simulink model "Clutch"  (R2020a)
settings: Solver=VariableStepAuto  StartTime=0.0  StopTime=10.0  RelTol=1e-3
undefined symbols (not defined in the file or in its folder): be, bv, Ie, Iv, R, uk, us
settings Model: DataDictionary=Clutch_lockup.sldd  Creator=USER  LastModifiedBy=USER

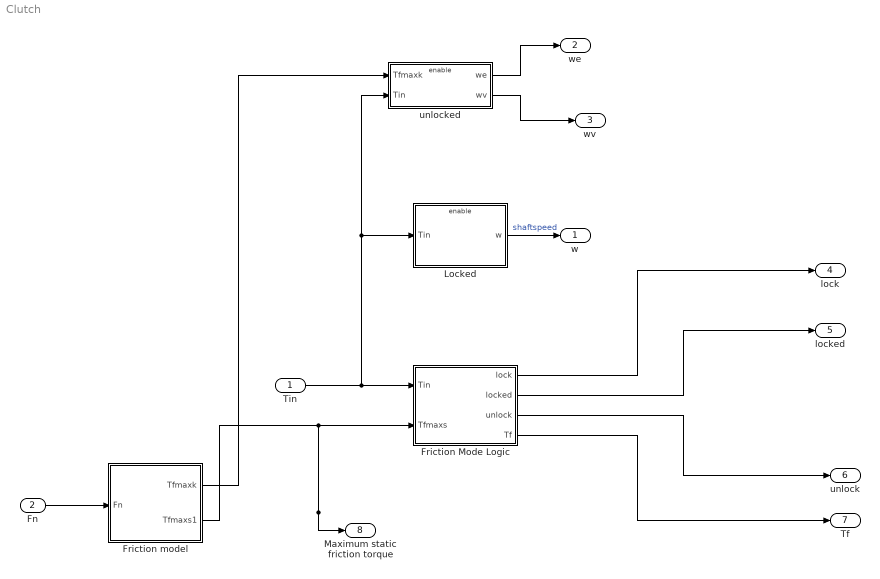
== system Clutch ==
  Tin : Inport
  Fn : Inport  Port=2
  Friction Mode Logic : Subsystem
  Friction model : Subsystem
  Locked : Subsystem
  unlocked : Subsystem
  w : Outport
  we : Outport  Port=2
  wv : Outport  Port=3
  lock : Outport  Port=4
  locked : Outport  Port=5
  unlock : Outport  Port=6
  Tf : Outport  Port=7
  Maximum static friction torque : Outport  Port=8
  wires:
  Locked/1(w) -> w/1  "shaftspeed"
  unlocked/1(we) -> we/1
  unlocked/2(wv) -> wv/1
  Friction model/2(Tfmaxs1) -> Maximum static friction torque/1, Friction Mode Logic/2(Tfmaxs)
  Tin/1 -> unlocked/2(Tin), Locked/1(Tin), Friction Mode Logic/1(Tin)
  Friction Mode Logic/1(lock) -> lock/1
  Friction Mode Logic/2(locked) -> locked/1
  Friction Mode Logic/3(unlock) -> unlock/1
  Friction Mode Logic/4(Tf) -> Tf/1
  Fn/1 -> Friction model/1(Fn)
  Friction model/1(Tfmaxk) -> unlocked/1(Tfmaxk)

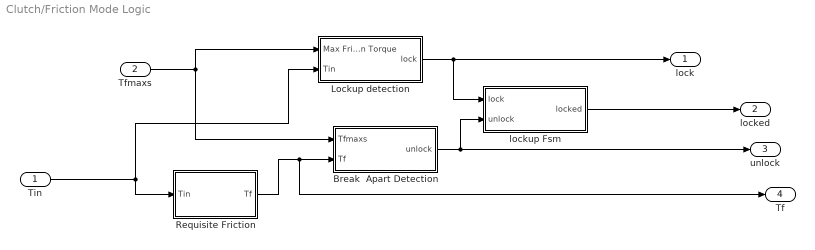
== system Clutch/Friction Mode Logic ==
  Tin : Inport
  Tfmaxs : Inport  Port=2
  Break  Apart Detection : Subsystem
  Lockup detection : Subsystem
  Requisite Friction : Subsystem
  lockup Fsm : Subsystem
  lock : Outport
  locked : Outport  Port=2
  unlock : Outport  Port=3
  Tf : Outport  Port=4
  wires:
  Lockup detection/1(lock) -> lock/1, lockup Fsm/1(lock)
  Requisite Friction/1(Tf) -> Tf/1, Break  Apart Detection/2(Tf)
  Tin/1 -> Lockup detection/2(Tin), Requisite Friction/1(Tin)
  Break  Apart Detection/1(unlock) -> unlock/1, lockup Fsm/2(unlock)
  Tfmaxs/1 -> Break  Apart Detection/1(Tfmaxs), Lockup detection/1(Max Friction Torque)
  lockup Fsm/1(locked) -> locked/1

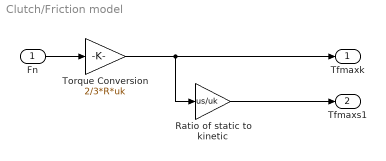
== system Clutch/Friction model ==
  Fn : Inport
  Ratio of static to kinetic : Gain  Gain=us/uk  SaturateOnIntegerOverflow=on  OutDataTypeStr=Inherit: Same as input  ParamDataTypeStr=Inherit: Same as input
  Torque Conversion : Gain  Gain=2/3*R*uk  SaturateOnIntegerOverflow=on  OutDataTypeStr=Inherit: Same as input  ParamDataTypeStr=Inherit: Same as input
  Tfmaxk : Outport  InitialOutput=0  VectorParamsAs1DForOutWhenUnconnected=off
  Tfmaxs1 : Outport  Port=2  InitialOutput=0  VectorParamsAs1DForOutWhenUnconnected=off
  wires:
  Torque Conversion/1 -> Tfmaxk/1, Ratio of static to kinetic/1
  Ratio of static to kinetic/1 -> Tfmaxs1/1
  Fn/1 -> Torque Conversion/1

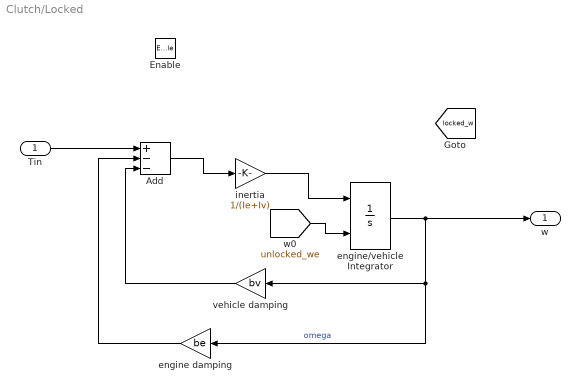
== system Clutch/Locked ==
  Tin : Inport
  Enable : EnablePort  StatesWhenEnabling=reset
  Add : Sum  Inputs=+--
  engine damping : Gain  Gain=be
  engine/vehicle Integrator : Integrator  InitialConditionSource=external
  inertia : Gain  Gain=1/(Ie+Iv)
  vehicle damping : Gain  Gain=bv
  w : Outport
  tag scope: locked_w=global
  wires:
  Add/1 -> inertia/1
  engine/vehicle Integrator/1 -> w/1, engine damping/1, vehicle damping/1  "omega"
  vehicle damping/1 -> Add/3
  Tin/1 -> Add/1
  engine damping/1 -> Add/2
  [unlocked_we] -> engine/vehicle Integrator/2
  inertia/1 -> engine/vehicle Integrator/1

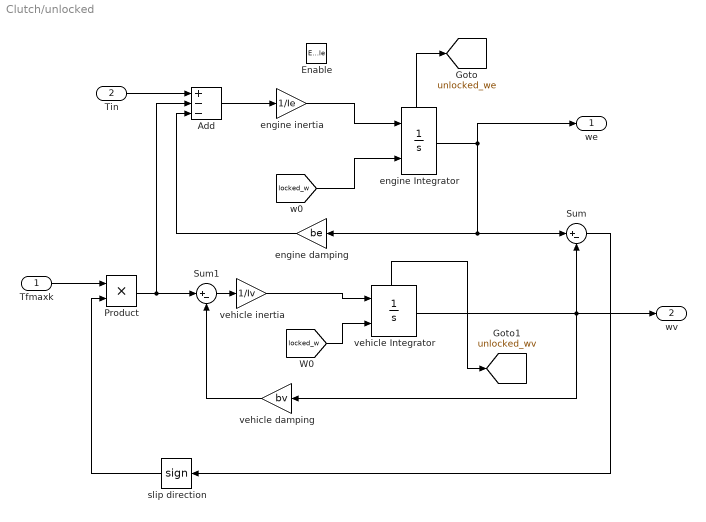
== system Clutch/unlocked ==
  Tfmaxk : Inport
  Tin : Inport  Port=2
  Enable : EnablePort  StatesWhenEnabling=reset
  Add : Sum  Inputs=+--
  Product : Product
  Sum : Sum  Inputs=|+-
  Sum1 : Sum  Inputs=|+-
  engine Integrator : Integrator  InitialConditionSource=external  ShowStatePort=on
  engine damping : Gain  Gain=be
  engine inertia : Gain  Gain=1/Ie
  slip direction : Signum
  vehicle Integrator : Integrator  InitialConditionSource=external  ShowStatePort=on
  vehicle damping : Gain  Gain=bv
  vehicle inertia : Gain  Gain=1/Iv
  we : Outport
  wv : Outport  Port=2
  tag scope: unlocked_we=global, unlocked_wv=global
  wires:
  Add/1 -> engine inertia/1
  engine inertia/1 -> engine Integrator/1
  engine Integrator/1 -> we/1, Sum/1, engine damping/1
  engine damping/1 -> Add/3
  [locked_w] -> engine Integrator/2
  Tin/1 -> Add/1
  Tfmaxk/1 -> Product/1
  Product/1 -> Sum1/1, Add/2
  Sum1/1 -> vehicle inertia/1
  vehicle damping/1 -> Sum1/2
  vehicle inertia/1 -> vehicle Integrator/1
  [locked_w] -> vehicle Integrator/2
  vehicle Integrator/1 -> Sum/2, vehicle damping/1, wv/1
  vehicle Integrator/State -> [unlocked_wv]
  slip direction/1 -> Product/2
  Sum/1 -> slip direction/1
  engine Integrator/State -> [unlocked_we]

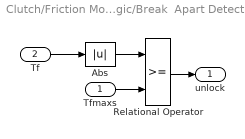
== system Clutch/Friction Mode Logic/Break  Apart Detection ==
  Tfmaxs : Inport
  Tf : Inport  Port=2
  Abs : Abs  SaturateOnIntegerOverflow=on
  Relational Operator : RelationalOperator  OutDataTypeStr=boolean  RndMeth=Nearest  InputSameDT=on
  unlock : Outport  InitialOutput=0  VectorParamsAs1DForOutWhenUnconnected=off
  wires:
  Tfmaxs/1 -> Relational Operator/2
  Tf/1 -> Abs/1
  Abs/1 -> Relational Operator/1
  Relational Operator/1 -> unlock/1

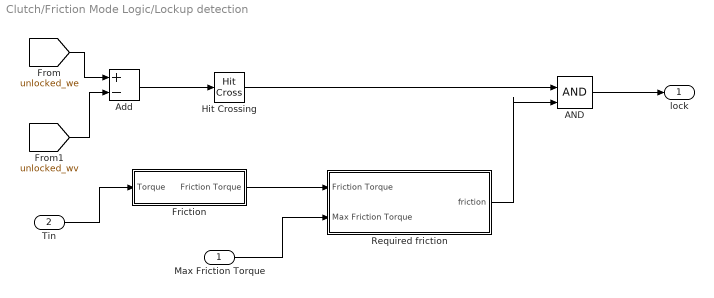
== system Clutch/Friction Mode Logic/Lockup detection ==
  Max Friction Torque : Inport
  Tin : Inport  Port=2
  AND : Logic  IconShape=distinctive  AllPortsSameDT=off  OutDataTypeStr=boolean
  Add : Sum  Inputs=+-
  Friction : Subsystem
  Hit Crossing : HitCross
  Required friction : Subsystem
  lock : Outport
  wires:
  Required friction/1(friction) -> AND/2
  Max Friction Torque/1 -> Required friction/2(Max Friction Torque)
  Friction/1(Friction Torque) -> Required friction/1(Friction Torque)
  [unlocked_we] -> Add/1
  [unlocked_wv] -> Add/2
  Add/1 -> Hit Crossing/1
  Hit Crossing/1 -> AND/1
  AND/1 -> lock/1
  Tin/1 -> Friction/1(Torque)

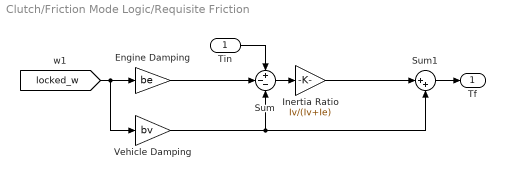
== system Clutch/Friction Mode Logic/Requisite Friction ==
  Tin : Inport
  Engine Damping : Gain  Gain=be  SaturateOnIntegerOverflow=on  OutDataTypeStr=Inherit: Same as input  ParamDataTypeStr=Inherit: Same as input
  Inertia Ratio : Gain  Gain=Iv/(Iv+Ie)  SaturateOnIntegerOverflow=on  OutDataTypeStr=Inherit: Same as input  ParamDataTypeStr=Inherit: Same as input
  Sum : Sum  Inputs=+--  InputSameDT=on  SaturateOnIntegerOverflow=on  OutDataTypeStr=Inherit: Same as first input
  Sum1 : Sum  Inputs=|++  InputSameDT=on  SaturateOnIntegerOverflow=on  OutDataTypeStr=Inherit: Same as first input
  Vehicle Damping : Gain  Gain=bv  SaturateOnIntegerOverflow=on  OutDataTypeStr=Inherit: Same as input  ParamDataTypeStr=Inherit: Same as input
  Tf : Outport  InitialOutput=0  VectorParamsAs1DForOutWhenUnconnected=off
  wires:
  [locked_w] -> Vehicle Damping/1, Engine Damping/1
  Engine Damping/1 -> Sum/2
  Vehicle Damping/1 -> Sum/3, Sum1/2
  Sum/1 -> Inertia Ratio/1
  Tin/1 -> Sum/1
  Inertia Ratio/1 -> Sum1/1
  Sum1/1 -> Tf/1

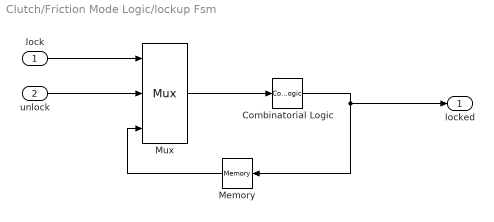
== system Clutch/Friction Mode Logic/lockup Fsm ==
  lock : Inport
  unlock : Inport  Port=2
  Combinatorial Logic : CombinatorialLogic  TruthTable=[0;1;0;0;1;1;1;0]
  Memory : Memory
  Mux : Mux  Inputs=3
  locked : Outport  InitialOutput=0  VectorParamsAs1DForOutWhenUnconnected=off
  wires:
  Combinatorial Logic/1 -> Memory/1, locked/1
  unlock/1 -> Mux/2
  lock/1 -> Mux/1
  Memory/1 -> Mux/3
  Mux/1 -> Combinatorial Logic/1

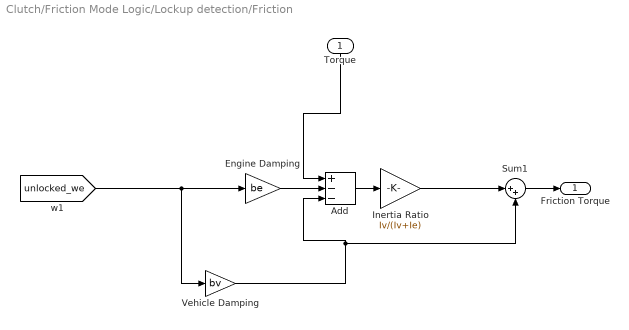
== system Clutch/Friction Mode Logic/Lockup detection/Friction ==
  Torque : Inport
  Add : Sum  Inputs=+--
  Engine Damping : Gain  Gain=be  SaturateOnIntegerOverflow=on  OutDataTypeStr=Inherit: Same as input  ParamDataTypeStr=Inherit: Same as input
  Inertia Ratio : Gain  Gain=Iv/(Iv+Ie)  SaturateOnIntegerOverflow=on  OutDataTypeStr=Inherit: Same as input  ParamDataTypeStr=Inherit: Same as input
  Sum1 : Sum  Inputs=|++  InputSameDT=on  SaturateOnIntegerOverflow=on  OutDataTypeStr=Inherit: Same as first input
  Vehicle Damping : Gain  Gain=bv  SaturateOnIntegerOverflow=on  OutDataTypeStr=Inherit: Same as input  ParamDataTypeStr=Inherit: Same as input
  Friction Torque : Outport  InitialOutput=0  VectorParamsAs1DForOutWhenUnconnected=off
  wires:
  [unlocked_we] -> Engine Damping/1, Vehicle Damping/1
  Vehicle Damping/1 -> Add/3, Sum1/2
  Engine Damping/1 -> Add/2
  Add/1 -> Inertia Ratio/1
  Torque/1 -> Add/1
  Inertia Ratio/1 -> Sum1/1
  Sum1/1 -> Friction Torque/1

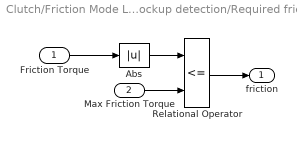
== system Clutch/Friction Mode Logic/Lockup detection/Required friction ==
  Friction Torque : Inport
  Max Friction Torque : Inport  Port=2
  Abs : Abs  SaturateOnIntegerOverflow=on
  Relational Operator : RelationalOperator  Operator=<=  OutDataTypeStr=boolean  RndMeth=Nearest  InputSameDT=on
  friction : Outport  InitialOutput=0  VectorParamsAs1DForOutWhenUnconnected=off
  wires:
  Friction Torque/1 -> Abs/1
  Relational Operator/1 -> friction/1
  Abs/1 -> Relational Operator/1
  Max Friction Torque/1 -> Relational Operator/2
